simulink model "HubDepotModel"  (Simulink 7.9)
settings: Solver=VariableStepDiscrete  StartTime=0.0  StopTime=100.0  RelTol=1e-3
undefined symbols (not defined in the file or in its folder): CustomerBase_1
libraries: simeventslib x10
(part 2 of 4)

== system HubDepotModel/Depot_3/Storage_Subsystem/<<SOURCE>> Source_Stocked_Product ==
  Output Switch : OutputSwitch  NumberOutputPorts=2
  Path Combiner : PathCombiner  NumberInputPorts=2
  Schedule_Product_Deliveries_CONTROL : Subsystem
  Transfer_Product_CONTROL : Subsystem
  sS1.1_Schedule_Product_Deliveries_PLANT : Subsystem
  sS1.2_Receive_Product_PLANT : Subsystem
  sS1.3_Transfer_Product_PLANT : Subsystem
  sS1.3_Verify_Product_PLANT : Subsystem
  Inventory_IN : PMIOPort  Port=1  Side=Left
  Inventory_OUT : PMIOPort  Port=2  Side=Right
  Replenishment_Shipment : PMIOPort  Port=3  Side=Left
  Replenishment_Signal : PMIOPort  Port=4  Side=Left
  Procurement_Order : PMIOPort  Port=5  Side=Right
  wires:
  Schedule_Product_Deliveries_CONTROL/3(Reorder_Signal) -> sS1.1_Schedule_Product_Deliveries_PLANT/3(Reorder_Signal)
  Schedule_Product_Deliveries_CONTROL/1(Component) -> sS1.1_Schedule_Product_Deliveries_PLANT/1(Component)
  Schedule_Product_Deliveries_CONTROL/2(Reorder_Quantity) -> sS1.1_Schedule_Product_Deliveries_PLANT/2(Reorder_Quantity)
  connections:
  Replenishment_Signal/RConn1 -- Schedule_Product_Deliveries_CONTROL/LConn2
  Path Combiner/LConn1 -- Schedule_Product_Deliveries_CONTROL/RConn1
  Path Combiner/LConn2 -- Transfer_Product_CONTROL/RConn1
  Path Combiner/RConn1 -- Inventory_OUT/RConn1
  Output Switch/RConn2 -- Transfer_Product_CONTROL/LConn1
  Output Switch/RConn1 -- Schedule_Product_Deliveries_CONTROL/LConn1
  Inventory_IN/RConn1 -- Output Switch/LConn1
  sS1.1_Schedule_Product_Deliveries_PLANT/RConn1 -- Procurement_Order/RConn1
  sS1.3_Transfer_Product_PLANT/RConn1 -- Transfer_Product_CONTROL/LConn2
  sS1.3_Verify_Product_PLANT/RConn1 -- sS1.3_Transfer_Product_PLANT/LConn1
  sS1.2_Receive_Product_PLANT/RConn1 -- sS1.3_Verify_Product_PLANT/LConn1
  Replenishment_Shipment/RConn1 -- sS1.2_Receive_Product_PLANT/LConn1

== system HubDepotModel/Depot_4/Storage_Subsystem/<<DELIVER>>Deliver_Stocked_Product ==
  Deliver_Stocked_Product_CONTROL : Subsystem
  sD1.10_Pack_Order_PLANT : Subsystem
  sD1.11_Load_Order_PLANT : Subsystem
  sD1.2_Receive_Order_PLANT : Subsystem
  sD1.4_Consolidate_Orders_PLANT : Subsystem
  sD1.9_Pick_Order_PLANT : Subsystem
  Inventory_IN : PMIOPort  Port=1  Side=Left
  Inventory_OUT : PMIOPort  Port=2  Side=Right
  Customer_Procurement_Order : PMIOPort  Port=3  Side=Left
  Fulfillment_Shipment : PMIOPort  Port=4  Side=Right
  Replenishment_Signal : PMIOPort  Port=5  Side=Right
  connections:
  sD1.4_Consolidate_Orders_PLANT/RConn1 -- sD1.9_Pick_Order_PLANT/LConn1
  sD1.2_Receive_Order_PLANT/RConn1 -- sD1.4_Consolidate_Orders_PLANT/LConn1
  Deliver_Stocked_Product_CONTROL/RConn2 -- Inventory_OUT/RConn1
  Deliver_Stocked_Product_CONTROL/RConn1 -- Replenishment_Signal/RConn1
  Deliver_Stocked_Product_CONTROL/LConn1 -- Inventory_IN/RConn1
  sD1.9_Pick_Order_PLANT/RConn1 -- Deliver_Stocked_Product_CONTROL/LConn2
  sD1.11_Load_Order_PLANT/RConn1 -- Fulfillment_Shipment/RConn1
  sD1.10_Pack_Order_PLANT/RConn1 -- sD1.11_Load_Order_PLANT/LConn1
  sD1.9_Pick_Order_PLANT/RConn2 -- sD1.10_Pack_Order_PLANT/LConn1
  Customer_Procurement_Order/RConn1 -- sD1.2_Receive_Order_PLANT/LConn1

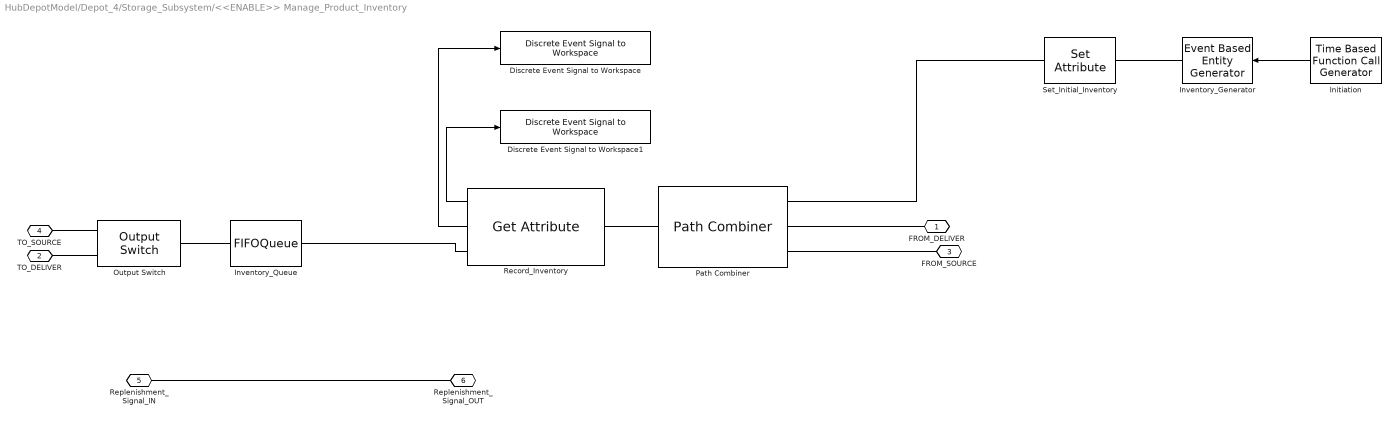
== system HubDepotModel/Depot_4/Storage_Subsystem/<<ENABLE>> Manage_Product_Inventory ==
  Discrete Event Signal to Workspace : simeventslib/SimEvents Sinks/Discrete Event Signal to Workspace  VariableName=Inventory_Position_Depot_1  SaveFormat=Structure With Time  isMonitorOnly=off  isRecordIC=off
  Discrete Event Signal to Workspace1 : simeventslib/SimEvents Sinks/Discrete Event Signal to Workspace  VariableName=Net_Inventory_Depot_1  SaveFormat=Structure With Time  isMonitorOnly=off  isRecordIC=off
  Initiation : TimeBasedFunctionCallGenerator  EventGenerationMode=Only at simulation start  EventPriority=1
  Inventory_Generator : EventBasedEntityGenerator  GenerateEntitiesUpon=Function call from port fcn  SpecifyEventPriority=on  PriorityEntityGeneration=1  AllowBlocking=off  EntityType=Standard
  Inventory_Queue : FIFOQueue
  Output Switch : OutputSwitch  NumberOutputPorts=2
  Path Combiner : PathCombiner
  Record_Inventory : GetAttribute  AttributeName=Net_Inventory|Inventory_Position  AttributeMissing=Error|Error  AttributeDefaultValue=1|1  AttributeTreatAsVector=1|1  AttributeSendTiming=After entity departure|After entity departure  EvaluatedDefaultAttributeValue={[];[]}
      settings: OutputPortMap=o1,o2
  Set_Initial_Inventory : SetAttribute  AttributeName=Net_Inventory|Inventory_Position|Reorder_Point|Reorder_Quantity  AttributeFrom=Dialog|Dialog|Dialog|Dialog  AttributeValue=[11 13]|[11 13]|[10 10]|[5 5]  AttributeTreatAsVector=1|1|1|1  EvaluatedAttributeValue={[11 13];[11 13];[10 10];[5 5]}
  FROM_DELIVER : PMIOPort  Port=1  Side=Left
  TO_DELIVER : PMIOPort  Port=2  Side=Right
  FROM_SOURCE : PMIOPort  Port=3  Side=Left
  TO_SOURCE : PMIOPort  Port=4  Side=Right
  Replenishment_Signal_IN : PMIOPort  Port=5  Side=Left
  Replenishment_Signal_OUT : PMIOPort  Port=6  Side=Right
  wires:
  Record_Inventory/2 -> Discrete Event Signal to Workspace/1
  Initiation/1 -> Inventory_Generator/1
  Record_Inventory/1 -> Discrete Event Signal to Workspace1/1
  connections:
  Set_Initial_Inventory/RConn1 -- Path Combiner/LConn1
  Replenishment_Signal_IN/RConn1 -- Replenishment_Signal_OUT/RConn1
  TO_SOURCE/RConn1 -- Output Switch/RConn1
  TO_DELIVER/RConn1 -- Output Switch/RConn2
  FROM_SOURCE/RConn1 -- Path Combiner/LConn3
  FROM_DELIVER/RConn1 -- Path Combiner/LConn2
  Record_Inventory/LConn1 -- Path Combiner/RConn1
  Output Switch/LConn1 -- Inventory_Queue/RConn1
  Record_Inventory/RConn1 -- Inventory_Queue/LConn1
  Set_Initial_Inventory/LConn1 -- Inventory_Generator/RConn1

== system HubDepotModel/Depot_4/Storage_Subsystem/<<SOURCE>> Source_Stocked_Product ==
  Output Switch : OutputSwitch  NumberOutputPorts=2
  Path Combiner : PathCombiner  NumberInputPorts=2
  Schedule_Product_Deliveries_CONTROL : Subsystem
  Transfer_Product_CONTROL : Subsystem
  sS1.1_Schedule_Product_Deliveries_PLANT : Subsystem
  sS1.2_Receive_Product_PLANT : Subsystem
  sS1.3_Transfer_Product_PLANT : Subsystem
  sS1.3_Verify_Product_PLANT : Subsystem
  Inventory_IN : PMIOPort  Port=1  Side=Left
  Inventory_OUT : PMIOPort  Port=2  Side=Right
  Replenishment_Shipment : PMIOPort  Port=3  Side=Left
  Replenishment_Signal : PMIOPort  Port=4  Side=Left
  Procurement_Order : PMIOPort  Port=5  Side=Right
  wires:
  Schedule_Product_Deliveries_CONTROL/3(Reorder_Signal) -> sS1.1_Schedule_Product_Deliveries_PLANT/3(Reorder_Signal)
  Schedule_Product_Deliveries_CONTROL/1(Component) -> sS1.1_Schedule_Product_Deliveries_PLANT/1(Component)
  Schedule_Product_Deliveries_CONTROL/2(Reorder_Quantity) -> sS1.1_Schedule_Product_Deliveries_PLANT/2(Reorder_Quantity)
  connections:
  Replenishment_Signal/RConn1 -- Schedule_Product_Deliveries_CONTROL/LConn2
  Path Combiner/LConn1 -- Schedule_Product_Deliveries_CONTROL/RConn1
  Path Combiner/LConn2 -- Transfer_Product_CONTROL/RConn1
  Path Combiner/RConn1 -- Inventory_OUT/RConn1
  Output Switch/RConn2 -- Transfer_Product_CONTROL/LConn1
  Output Switch/RConn1 -- Schedule_Product_Deliveries_CONTROL/LConn1
  Inventory_IN/RConn1 -- Output Switch/LConn1
  sS1.1_Schedule_Product_Deliveries_PLANT/RConn1 -- Procurement_Order/RConn1
  sS1.3_Transfer_Product_PLANT/RConn1 -- Transfer_Product_CONTROL/LConn2
  sS1.3_Verify_Product_PLANT/RConn1 -- sS1.3_Transfer_Product_PLANT/LConn1
  sS1.2_Receive_Product_PLANT/RConn1 -- sS1.3_Verify_Product_PLANT/LConn1
  Replenishment_Shipment/RConn1 -- sS1.2_Receive_Product_PLANT/LConn1

== system HubDepotModel/Hub_1/Storage_Subsystem/<<DELIVER>>Deliver_Stocked_Product ==
  Deliver_Stocked_Product_CONTROL : Subsystem
  sD1.10_Pack_Order_PLANT : Subsystem
  sD1.11_Load_Order_PLANT : Subsystem
  sD1.2_Receive_Order_PLANT : Subsystem
  sD1.4_Consolidate_Orders_PLANT : Subsystem
  sD1.9_Pick_Order_PLANT : Subsystem
  Inventory_IN : PMIOPort  Port=1  Side=Left
  Inventory_OUT : PMIOPort  Port=2  Side=Right
  Customer_Procurement_Order : PMIOPort  Port=3  Side=Left
  Fulfillment_Shipment : PMIOPort  Port=4  Side=Right
  Replenishment_Signal : PMIOPort  Port=5  Side=Right
  connections:
  sD1.4_Consolidate_Orders_PLANT/RConn1 -- sD1.9_Pick_Order_PLANT/LConn1
  sD1.2_Receive_Order_PLANT/RConn1 -- sD1.4_Consolidate_Orders_PLANT/LConn1
  Deliver_Stocked_Product_CONTROL/RConn2 -- Inventory_OUT/RConn1
  Deliver_Stocked_Product_CONTROL/RConn1 -- Replenishment_Signal/RConn1
  Deliver_Stocked_Product_CONTROL/LConn1 -- Inventory_IN/RConn1
  sD1.9_Pick_Order_PLANT/RConn1 -- Deliver_Stocked_Product_CONTROL/LConn2
  sD1.11_Load_Order_PLANT/RConn1 -- Fulfillment_Shipment/RConn1
  sD1.10_Pack_Order_PLANT/RConn1 -- sD1.11_Load_Order_PLANT/LConn1
  sD1.9_Pick_Order_PLANT/RConn2 -- sD1.10_Pack_Order_PLANT/LConn1
  Customer_Procurement_Order/RConn1 -- sD1.2_Receive_Order_PLANT/LConn1

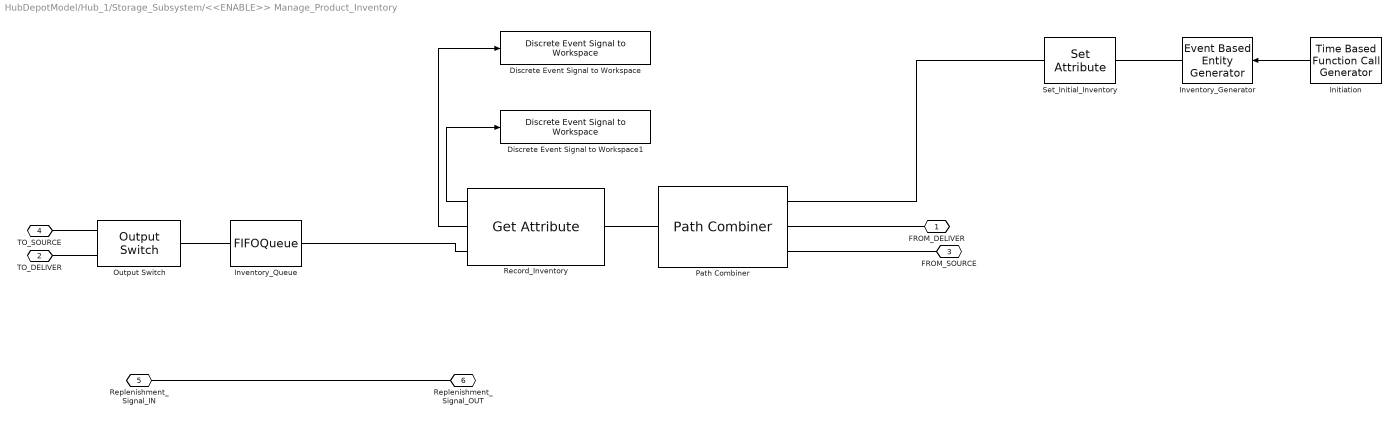
== system HubDepotModel/Hub_1/Storage_Subsystem/<<ENABLE>> Manage_Product_Inventory ==
  Discrete Event Signal to Workspace : simeventslib/SimEvents Sinks/Discrete Event Signal to Workspace  VariableName=Inventory_Position_Depot_1  SaveFormat=Structure With Time  isMonitorOnly=off  isRecordIC=off
  Discrete Event Signal to Workspace1 : simeventslib/SimEvents Sinks/Discrete Event Signal to Workspace  VariableName=Net_Inventory_Depot_1  SaveFormat=Structure With Time  isMonitorOnly=off  isRecordIC=off
  Initiation : TimeBasedFunctionCallGenerator  EventGenerationMode=Only at simulation start  EventPriority=1
  Inventory_Generator : EventBasedEntityGenerator  GenerateEntitiesUpon=Function call from port fcn  SpecifyEventPriority=on  PriorityEntityGeneration=1  AllowBlocking=off  EntityType=Standard
  Inventory_Queue : FIFOQueue
  Output Switch : OutputSwitch  NumberOutputPorts=2
  Path Combiner : PathCombiner
  Record_Inventory : GetAttribute  AttributeName=Net_Inventory|Inventory_Position  AttributeMissing=Error|Error  AttributeDefaultValue=1|1  AttributeTreatAsVector=1|1  AttributeSendTiming=After entity departure|After entity departure  EvaluatedDefaultAttributeValue={[];[]}
      settings: OutputPortMap=o1,o2
  Set_Initial_Inventory : SetAttribute  AttributeName=Net_Inventory|Inventory_Position|Reorder_Point|Reorder_Quantity  AttributeFrom=Dialog|Dialog|Dialog|Dialog  AttributeValue=[11 13]|[11 13]|[10 10]|[5 5]  AttributeTreatAsVector=1|1|1|1  EvaluatedAttributeValue={[11 13];[11 13];[10 10];[5 5]}
  FROM_DELIVER : PMIOPort  Port=1  Side=Left
  TO_DELIVER : PMIOPort  Port=2  Side=Right
  FROM_SOURCE : PMIOPort  Port=3  Side=Left
  TO_SOURCE : PMIOPort  Port=4  Side=Right
  Replenishment_Signal_IN : PMIOPort  Port=5  Side=Left
  Replenishment_Signal_OUT : PMIOPort  Port=6  Side=Right
  wires:
  Record_Inventory/2 -> Discrete Event Signal to Workspace/1
  Initiation/1 -> Inventory_Generator/1
  Record_Inventory/1 -> Discrete Event Signal to Workspace1/1
  connections:
  Set_Initial_Inventory/RConn1 -- Path Combiner/LConn1
  Replenishment_Signal_IN/RConn1 -- Replenishment_Signal_OUT/RConn1
  TO_SOURCE/RConn1 -- Output Switch/RConn1
  TO_DELIVER/RConn1 -- Output Switch/RConn2
  FROM_SOURCE/RConn1 -- Path Combiner/LConn3
  FROM_DELIVER/RConn1 -- Path Combiner/LConn2
  Record_Inventory/LConn1 -- Path Combiner/RConn1
  Output Switch/LConn1 -- Inventory_Queue/RConn1
  Record_Inventory/RConn1 -- Inventory_Queue/LConn1
  Set_Initial_Inventory/LConn1 -- Inventory_Generator/RConn1

== system HubDepotModel/Hub_1/Storage_Subsystem/<<SOURCE>> Source_Stocked_Product ==
  Output Switch : OutputSwitch  NumberOutputPorts=2
  Path Combiner : PathCombiner  NumberInputPorts=2
  Schedule_Product_Deliveries_CONTROL : Subsystem
  Transfer_Product_CONTROL : Subsystem
  sS1.1_Schedule_Product_Deliveries_PLANT : Subsystem
  sS1.2_Receive_Product_PLANT : Subsystem
  sS1.3_Transfer_Product_PLANT : Subsystem
  sS1.3_Verify_Product_PLANT : Subsystem
  Inventory_IN : PMIOPort  Port=1  Side=Left
  Inventory_OUT : PMIOPort  Port=2  Side=Right
  Replenishment_Shipment : PMIOPort  Port=3  Side=Left
  Replenishment_Signal : PMIOPort  Port=4  Side=Left
  Procurement_Order : PMIOPort  Port=5  Side=Right
  wires:
  Schedule_Product_Deliveries_CONTROL/3(Reorder_Signal) -> sS1.1_Schedule_Product_Deliveries_PLANT/3(Reorder_Signal)
  Schedule_Product_Deliveries_CONTROL/1(Component) -> sS1.1_Schedule_Product_Deliveries_PLANT/1(Component)
  Schedule_Product_Deliveries_CONTROL/2(Reorder_Quantity) -> sS1.1_Schedule_Product_Deliveries_PLANT/2(Reorder_Quantity)
  connections:
  Replenishment_Signal/RConn1 -- Schedule_Product_Deliveries_CONTROL/LConn2
  Path Combiner/LConn1 -- Schedule_Product_Deliveries_CONTROL/RConn1
  Path Combiner/LConn2 -- Transfer_Product_CONTROL/RConn1
  Path Combiner/RConn1 -- Inventory_OUT/RConn1
  Output Switch/RConn2 -- Transfer_Product_CONTROL/LConn1
  Output Switch/RConn1 -- Schedule_Product_Deliveries_CONTROL/LConn1
  Inventory_IN/RConn1 -- Output Switch/LConn1
  sS1.1_Schedule_Product_Deliveries_PLANT/RConn1 -- Procurement_Order/RConn1
  sS1.3_Transfer_Product_PLANT/RConn1 -- Transfer_Product_CONTROL/LConn2
  sS1.3_Verify_Product_PLANT/RConn1 -- sS1.3_Transfer_Product_PLANT/LConn1
  sS1.2_Receive_Product_PLANT/RConn1 -- sS1.3_Verify_Product_PLANT/LConn1
  Replenishment_Shipment/RConn1 -- sS1.2_Receive_Product_PLANT/LConn1

== system HubDepotModel/Depot_1/Storage_Subsystem/<<DELIVER>>Deliver_Stocked_Product/Deliver_Stocked_Product_CONTROL ==
  Calculate_Inventory_C : MATLAB Function  TreatAsAtomicUnit=on
  Combine_Consumption_Inventory : EntityCombiner  NumberInputPorts=2
  Consumption_Attributes : GetAttribute  AttributeName=Component|Consumption_Quantity|Net_Inventory|Inventory_Position  AttributeMissing=Error|Error|Error|Error  AttributeDefaultValue=1|1|1|1  AttributeTreatAsVector=1|1|1|1  AttributeSendTiming=After entity departure|After entity departure|After entity departure|After entity departure  EvaluatedDefaultAttributeValue={[];[];[];[]}
      settings: OutputPortMap=o1,o2,o3,o4
  Consumption_Server : SingleServer  ServiceTime=0
  Consumption_Sink : EntitySink
  FIFO Queue : FIFOQueue
  Replicate : Replicate  NumberOutputPorts=2
  Return_Inventory : EntitySplitter  NumberOutputPorts=2
  Set_Inventory_Level : SetAttribute  AttributeName=Net_Inventory|Inventory_Position  AttributeFrom=Signal port|Signal port  AttributeValue=1|1  AttributeTreatAsVector=1|1  EvaluatedAttributeValue={[];[]}
      settings: InputPortMap=u0,u1
  Inventory_IN : PMIOPort  Port=1  Side=Left
  Consumption_Signal_IN : PMIOPort  Port=2  Side=Left
  Consumption_Signal_OUT : PMIOPort  Port=3  Side=Right
  Inventory_OUT : PMIOPort  Port=4  Side=Right
  wires:
  Calculate_Inventory_C/2(out_Inventory_Position) -> Set_Inventory_Level/2
  Consumption_Attributes/4 -> Calculate_Inventory_C/2(Inventory_Position)
  Consumption_Attributes/2 -> Calculate_Inventory_C/4(Consumption_Quantity)
  Consumption_Attributes/3 -> Calculate_Inventory_C/1(Net_Inventory)
  Calculate_Inventory_C/1(out_Net_Inventory) -> Set_Inventory_Level/1
  Consumption_Attributes/1 -> Calculate_Inventory_C/3(Component)
  connections:
  Inventory_OUT/RConn1 -- Return_Inventory/RConn1
  Set_Inventory_Level/RConn1 -- Return_Inventory/LConn1
  Replicate/RConn2 -- Consumption_Signal_OUT/RConn1
  Return_Inventory/RConn2 -- Consumption_Sink/LConn1
  Consumption_Server/RConn1 -- Set_Inventory_Level/LConn1
  Consumption_Attributes/RConn1 -- Consumption_Server/LConn1
  Combine_Consumption_Inventory/RConn1 -- Consumption_Attributes/LConn1
  Replicate/RConn1 -- Combine_Consumption_Inventory/LConn2
  Inventory_IN/RConn1 -- Combine_Consumption_Inventory/LConn1
  Consumption_Signal_IN/RConn1 -- FIFO Queue/LConn1
  FIFO Queue/RConn1 -- Replicate/LConn1

== system HubDepotModel/Depot_1/Storage_Subsystem/<<DELIVER>>Deliver_Stocked_Product/sD1.10_Pack_Order_PLANT ==
  Entity Departure Function-Call Generator : EntityDepartureFunctionCallGenerator
  Event-Based Entity Generator : EventBasedEntityGenerator  GenerateEntitiesUpon=Function call from port fcn
  Get_Order_Attribute : GetAttribute  AttributeName=Component|Order_Quantity|Customer  AttributeMissing=Error|Error|Error  AttributeDefaultValue=1|1|1  AttributeTreatAsVector=1|1|1  AttributeSendTiming=After entity departure|After entity departure|After entity departure  EvaluatedDefaultAttributeValue={[];[];[]}
      settings: OutputPortMap=o1,o2,o3
  Order_Sink : EntitySink
  Set_Shipment_Attributes : SetAttribute  AttributeName=Component|Shipment_Quantity|Customer  AttributeFrom=Signal port|Signal port|Signal port  AttributeValue=1|1|1  AttributeTreatAsVector=1|1|1  EvaluatedAttributeValue={[];[];[]}
      settings: InputPortMap=u0,u1,u2
  sD1.10_Queue : FIFOQueue
  sD1.10_Server : NServer  NumberOfServers=inf  ServiceTime=0
  Order_IN : PMIOPort  Port=1  Side=Left
  Shipment_OUT : PMIOPort  Port=2  Side=Right
  wires:
  Get_Order_Attribute/3 -> Set_Shipment_Attributes/3
  Get_Order_Attribute/1 -> Set_Shipment_Attributes/1
  Get_Order_Attribute/2 -> Set_Shipment_Attributes/2
  Entity Departure Function-Call Generator/1 -> Event-Based Entity Generator/1
  connections:
  Get_Order_Attribute/RConn1 -- Entity Departure Function-Call Generator/LConn1
  sD1.10_Server/RConn1 -- Get_Order_Attribute/LConn1
  Order_Sink/LConn1 -- Entity Departure Function-Call Generator/RConn1
  Set_Shipment_Attributes/RConn1 -- Shipment_OUT/RConn1
  Event-Based Entity Generator/RConn1 -- Set_Shipment_Attributes/LConn1
  Order_IN/RConn1 -- sD1.10_Queue/LConn1
  sD1.10_Queue/RConn1 -- sD1.10_Server/LConn1

== system HubDepotModel/Depot_1/Storage_Subsystem/<<DELIVER>>Deliver_Stocked_Product/sD1.11_Load_Order_PLANT ==
  sD1.11_Queue : FIFOQueue
  sD1.11_Server : NServer  NumberOfServers=inf  ServiceTime=0
  Shipment_IN : PMIOPort  Port=1  Side=Left
  Shipment_OUT : PMIOPort  Port=2  Side=Right
  connections:
  Shipment_OUT/RConn1 -- sD1.11_Server/RConn1
  Shipment_IN/RConn1 -- sD1.11_Queue/LConn1
  sD1.11_Queue/RConn1 -- sD1.11_Server/LConn1

== system HubDepotModel/Depot_1/Storage_Subsystem/<<DELIVER>>Deliver_Stocked_Product/sD1.2_Receive_Order_PLANT ==
  sD1.2_Queue : FIFOQueue
  sD1.2_Server : NServer  NumberOfServers=inf  ServiceTime=0
  Order_IN : PMIOPort  Port=1  Side=Left
  Order_OUT : PMIOPort  Port=2  Side=Right
  connections:
  Order_OUT/RConn1 -- sD1.2_Server/RConn1
  Order_IN/RConn1 -- sD1.2_Queue/LConn1
  sD1.2_Queue/RConn1 -- sD1.2_Server/LConn1

== system HubDepotModel/Depot_1/Storage_Subsystem/<<DELIVER>>Deliver_Stocked_Product/sD1.4_Consolidate_Orders_PLANT ==
  sD1.4_Queue : FIFOQueue
  sD1.4_Server : NServer  NumberOfServers=inf  ServiceTime=0
  Order_IN : PMIOPort  Port=1  Side=Left
  Order_OUT : PMIOPort  Port=2  Side=Right
  connections:
  Order_OUT/RConn1 -- sD1.4_Server/RConn1
  Order_IN/RConn1 -- sD1.4_Queue/LConn1
  sD1.4_Queue/RConn1 -- sD1.4_Server/LConn1

== system HubDepotModel/Depot_1/Storage_Subsystem/<<DELIVER>>Deliver_Stocked_Product/sD1.9_Pick_Order_PLANT ==
  Generate_Consumption_Signal : Subsystem
  sD1.9_Queue : FIFOQueue
  sD1.9_Server : NServer  NumberOfServers=inf  ServiceTime=0
  Order_IN : PMIOPort  Port=1  Side=Left
  Consumption_Signal : PMIOPort  Port=2  Side=Right
  Order_OUT : PMIOPort  Port=3  Side=Right
  connections:
  Generate_Consumption_Signal/RConn2 -- Consumption_Signal/RConn1
  Generate_Consumption_Signal/RConn1 -- Order_OUT/RConn1
  sD1.9_Server/RConn1 -- Generate_Consumption_Signal/LConn1
  Order_IN/RConn1 -- sD1.9_Queue/LConn1
  sD1.9_Queue/RConn1 -- sD1.9_Server/LConn1

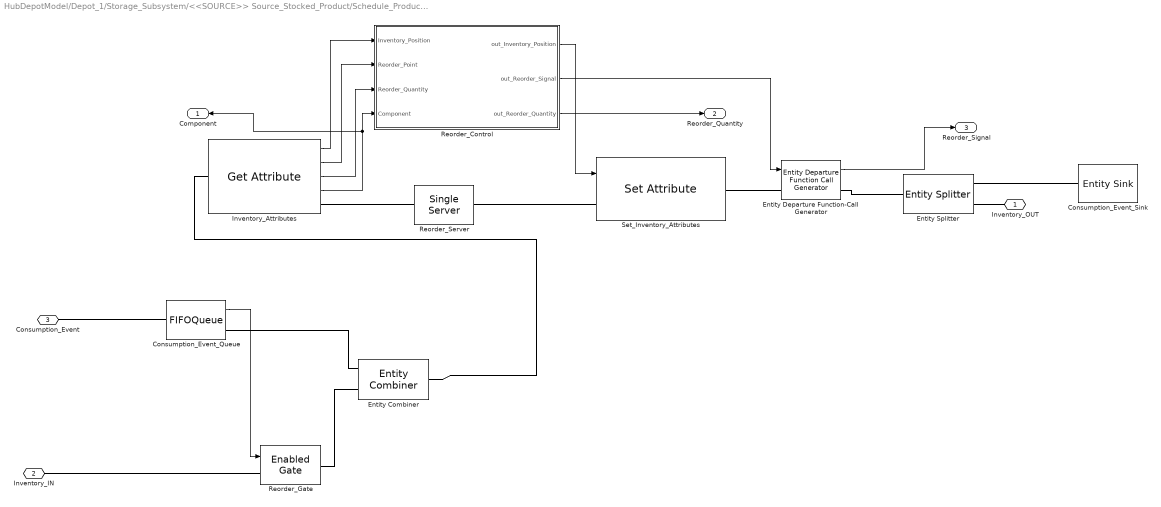
== system HubDepotModel/Depot_1/Storage_Subsystem/<<SOURCE>> Source_Stocked_Product/Schedule_Product_Deliveries_CONTROL ==
  Consumption_Event_Queue : FIFOQueue  StatNumberInBlock=on
      settings: OutputPortMap=o1
  Consumption_Event_Sink : EntitySink
  Entity Combiner : EntityCombiner  NumberInputPorts=2
  Entity Departure Function-Call Generator : EntityDepartureFunctionCallGenerator  EnableE1Port=on
  Entity Splitter : EntitySplitter  NumberOutputPorts=2
  Inventory_Attributes : GetAttribute  AttributeName=Inventory_Position|Reorder_Point|Reorder_Quantity|Component  AttributeMissing=Error|Error|Error|Error  AttributeDefaultValue=1|1|1|1  AttributeTreatAsVector=1|1|1|1  AttributeSendTiming=After entity departure|After entity departure|After entity departure|After entity departure  EvaluatedDefaultAttributeValue={[];[];[];[]}
      settings: OutputPortMap=o1,o2,o3,o4
  Reorder_Control : MATLAB Function  TreatAsAtomicUnit=on
  Reorder_Gate : EnabledGate
  Reorder_Server : SingleServer  ServiceTime=0
  Set_Inventory_Attributes : SetAttribute  AttributeName=Inventory_Position  AttributeFrom=Signal port  EvaluatedAttributeValue={[]}
  Inventory_OUT : PMIOPort  Port=1  Side=Right
  Inventory_IN : PMIOPort  Port=2  Side=Left
  Consumption_Event : PMIOPort  Port=3  Side=Left
  Component : Outport
  Reorder_Quantity : Outport  Port=2
  Reorder_Signal : Outport  Port=3
  wires:
  Entity Departure Function-Call Generator/1 -> Reorder_Signal/1
  Reorder_Control/3(out_Reorder_Quantity) -> Reorder_Quantity/1
  Consumption_Event_Queue/1 -> Reorder_Gate/1
  Reorder_Control/2(out_Reorder_Signal) -> Entity Departure Function-Call Generator/1
  Inventory_Attributes/4 -> Component/1, Reorder_Control/4(Component)
  Reorder_Control/1(out_Inventory_Position) -> Set_Inventory_Attributes/1
  Inventory_Attributes/3 -> Reorder_Control/3(Reorder_Quantity)
  Inventory_Attributes/2 -> Reorder_Control/2(Reorder_Point)
  Inventory_Attributes/1 -> Reorder_Control/1(Inventory_Position)
  connections:
  Entity Departure Function-Call Generator/RConn1 -- Entity Splitter/LConn1
  Set_Inventory_Attributes/RConn1 -- Entity Departure Function-Call Generator/LConn1
  Reorder_Server/RConn1 -- Set_Inventory_Attributes/LConn1
  Inventory_IN/RConn1 -- Reorder_Gate/LConn1
  Inventory_Attributes/RConn1 -- Reorder_Server/LConn1
  Inventory_OUT/RConn1 -- Entity Splitter/RConn2
  Entity Combiner/RConn1 -- Inventory_Attributes/LConn1
  Reorder_Gate/RConn1 -- Entity Combiner/LConn2
  Entity Splitter/RConn1 -- Consumption_Event_Sink/LConn1
  Consumption_Event_Queue/RConn1 -- Entity Combiner/LConn1
  Consumption_Event/RConn1 -- Consumption_Event_Queue/LConn1

== system HubDepotModel/Depot_1/Storage_Subsystem/<<SOURCE>> Source_Stocked_Product/Transfer_Product_CONTROL ==
  Calculate_Inventory : MATLAB Function  TreatAsAtomicUnit=on
  Combine_Inventory_and_Availability : EntityCombiner  NumberInputPorts=2
  FIFO Queue : FIFOQueue
  Inventory_Availability_Attributes : GetAttribute  AttributeName=Component|Shipment_Quantity|Net_Inventory  AttributeMissing=Error|Error|Error  AttributeDefaultValue=1|1|1  AttributeTreatAsVector=1|1|1  AttributeSendTiming=After entity departure|After entity departure|After entity departure  EvaluatedDefaultAttributeValue={[];[];[]}
      settings: OutputPortMap=o1,o2,o3
  Inventory_Availability_Sink : EntitySink
  Return_Inventory : EntitySplitter  NumberOutputPorts=2
  Server : SingleServer  ServiceTime=0
  Set_Inventory_Level : SetAttribute  AttributeName=Net_Inventory  AttributeFrom=Signal port  EvaluatedAttributeValue={[]}
  Inventory_OUT : PMIOPort  Port=1  Side=Right
  Inventory_IN : PMIOPort  Port=2  Side=Left
  Inventory_Availability_Signal : PMIOPort  Port=3  Side=Left
  wires:
  Inventory_Availability_Attributes/2 -> Calculate_Inventory/3(Shipment_Quantity)
  Inventory_Availability_Attributes/3 -> Calculate_Inventory/1(Net_Inventory)
  Calculate_Inventory/1(out_Inventory) -> Set_Inventory_Level/1
  Inventory_Availability_Attributes/1 -> Calculate_Inventory/2(Component)
  connections:
  Inventory_IN/RConn1 -- Combine_Inventory_and_Availability/LConn1
  FIFO Queue/RConn1 -- Combine_Inventory_and_Availability/LConn2
  Inventory_Availability_Signal/RConn1 -- FIFO Queue/LConn1
  Inventory_OUT/RConn1 -- Return_Inventory/RConn1
  Set_Inventory_Level/RConn1 -- Return_Inventory/LConn1
  Return_Inventory/RConn2 -- Inventory_Availability_Sink/LConn1
  Server/RConn1 -- Set_Inventory_Level/LConn1
  Inventory_Availability_Attributes/RConn1 -- Server/LConn1
  Combine_Inventory_and_Availability/RConn1 -- Inventory_Availability_Attributes/LConn1

== system HubDepotModel/Depot_1/Storage_Subsystem/<<SOURCE>> Source_Stocked_Product/sS1.1_Schedule_Product_Deliveries_PLANT ==
  Component : Inport
  Reorder_Quantity : Inport  Port=2
  Reorder_Signal : Inport  Port=3
  Generate_Procurement_Order : Subsystem
  Schedule_Product_Deliveries_Server : NServer  NumberOfServers=inf  ServiceTime=0
  Set_Procurement_Order : SetAttribute  AttributeName=Component|Order_Quantity|Supplier|Customer  AttributeFrom=Signal port|Signal port|Dialog|Dialog  AttributeValue=1|1|1|1  AttributeTreatAsVector=1|1|1|1  EvaluatedAttributeValue={[];[];1;1}
      settings: InputPortMap=u0,u1
  Procurement_Order : PMIOPort  Port=1  Side=Right
  wires:
  Reorder_Signal/1 -> Generate_Procurement_Order/1(Reorder_Signal)
  Reorder_Quantity/1 -> Set_Procurement_Order/2
  Component/1 -> Set_Procurement_Order/1
  connections:
  Procurement_Order/RConn1 -- Set_Procurement_Order/RConn1
  Schedule_Product_Deliveries_Server/RConn1 -- Set_Procurement_Order/LConn1
  Generate_Procurement_Order/RConn1 -- Schedule_Product_Deliveries_Server/LConn1

== system HubDepotModel/Depot_1/Storage_Subsystem/<<SOURCE>> Source_Stocked_Product/sS1.2_Receive_Product_PLANT ==
  sS1.2_Queue : FIFOQueue  Capacity=inf
  sS1.2_Server : NServer  NumberOfServers=inf  ServiceTime=0
  Shipment_IN : PMIOPort  Port=1  Side=Left
  Component_OUT : PMIOPort  Port=2  Side=Right
  connections:
  Component_OUT/RConn1 -- sS1.2_Server/RConn1
  Shipment_IN/RConn1 -- sS1.2_Queue/LConn1
  sS1.2_Queue/RConn1 -- sS1.2_Server/LConn1

== system HubDepotModel/Depot_1/Storage_Subsystem/<<SOURCE>> Source_Stocked_Product/sS1.3_Transfer_Product_PLANT ==
  sS1.4_Queue : FIFOQueue
  sS1.4_Server : NServer  NumberOfServers=inf  ServiceTime=0
  Component_IN : PMIOPort  Port=1  Side=Left
  Inventory_Availability_Signal : PMIOPort  Port=2  Side=Right
  connections:
  Inventory_Availability_Signal/RConn1 -- sS1.4_Server/RConn1
  Component_IN/RConn1 -- sS1.4_Queue/LConn1
  sS1.4_Queue/RConn1 -- sS1.4_Server/LConn1

== system HubDepotModel/Depot_1/Storage_Subsystem/<<SOURCE>> Source_Stocked_Product/sS1.3_Verify_Product_PLANT ==
  sS1.3_Queue : FIFOQueue  Capacity=inf
  sS1.3_Server : NServer  NumberOfServers=inf  ServiceTime=0
  Component_IN : PMIOPort  Port=1  Side=Left
  Component_OUT : PMIOPort  Port=2  Side=Right
  connections:
  Component_OUT/RConn1 -- sS1.3_Server/RConn1
  Component_IN/RConn1 -- sS1.3_Queue/LConn1
  sS1.3_Queue/RConn1 -- sS1.3_Server/LConn1

== system HubDepotModel/Depot_2/Storage_Subsystem/<<DELIVER>>Deliver_Stocked_Product/Deliver_Stocked_Product_CONTROL ==
  Calculate_Inventory_C : MATLAB Function  TreatAsAtomicUnit=on
  Combine_Consumption_Inventory : EntityCombiner  NumberInputPorts=2
  Consumption_Attributes : GetAttribute  AttributeName=Component|Consumption_Quantity|Net_Inventory|Inventory_Position  AttributeMissing=Error|Error|Error|Error  AttributeDefaultValue=1|1|1|1  AttributeTreatAsVector=1|1|1|1  AttributeSendTiming=After entity departure|After entity departure|After entity departure|After entity departure  EvaluatedDefaultAttributeValue={[];[];[];[]}
      settings: OutputPortMap=o1,o2,o3,o4
  Consumption_Server : SingleServer  ServiceTime=0
  Consumption_Sink : EntitySink
  FIFO Queue : FIFOQueue
  Replicate : Replicate  NumberOutputPorts=2
  Return_Inventory : EntitySplitter  NumberOutputPorts=2
  Set_Inventory_Level : SetAttribute  AttributeName=Net_Inventory|Inventory_Position  AttributeFrom=Signal port|Signal port  AttributeValue=1|1  AttributeTreatAsVector=1|1  EvaluatedAttributeValue={[];[]}
      settings: InputPortMap=u0,u1
  Inventory_IN : PMIOPort  Port=1  Side=Left
  Consumption_Signal_IN : PMIOPort  Port=2  Side=Left
  Consumption_Signal_OUT : PMIOPort  Port=3  Side=Right
  Inventory_OUT : PMIOPort  Port=4  Side=Right
  wires:
  Calculate_Inventory_C/2(out_Inventory_Position) -> Set_Inventory_Level/2
  Consumption_Attributes/4 -> Calculate_Inventory_C/2(Inventory_Position)
  Consumption_Attributes/2 -> Calculate_Inventory_C/4(Consumption_Quantity)
  Consumption_Attributes/3 -> Calculate_Inventory_C/1(Net_Inventory)
  Calculate_Inventory_C/1(out_Net_Inventory) -> Set_Inventory_Level/1
  Consumption_Attributes/1 -> Calculate_Inventory_C/3(Component)
  connections:
  Inventory_OUT/RConn1 -- Return_Inventory/RConn1
  Set_Inventory_Level/RConn1 -- Return_Inventory/LConn1
  Replicate/RConn2 -- Consumption_Signal_OUT/RConn1
  Return_Inventory/RConn2 -- Consumption_Sink/LConn1
  Consumption_Server/RConn1 -- Set_Inventory_Level/LConn1
  Consumption_Attributes/RConn1 -- Consumption_Server/LConn1
  Combine_Consumption_Inventory/RConn1 -- Consumption_Attributes/LConn1
  Replicate/RConn1 -- Combine_Consumption_Inventory/LConn2
  Inventory_IN/RConn1 -- Combine_Consumption_Inventory/LConn1
  Consumption_Signal_IN/RConn1 -- FIFO Queue/LConn1
  FIFO Queue/RConn1 -- Replicate/LConn1

== system HubDepotModel/Depot_2/Storage_Subsystem/<<DELIVER>>Deliver_Stocked_Product/sD1.10_Pack_Order_PLANT ==
  Entity Departure Function-Call Generator : EntityDepartureFunctionCallGenerator
  Event-Based Entity Generator : EventBasedEntityGenerator  GenerateEntitiesUpon=Function call from port fcn
  Get_Order_Attribute : GetAttribute  AttributeName=Component|Order_Quantity|Customer  AttributeMissing=Error|Error|Error  AttributeDefaultValue=1|1|1  AttributeTreatAsVector=1|1|1  AttributeSendTiming=After entity departure|After entity departure|After entity departure  EvaluatedDefaultAttributeValue={[];[];[]}
      settings: OutputPortMap=o1,o2,o3
  Order_Sink : EntitySink
  Set_Shipment_Attributes : SetAttribute  AttributeName=Component|Shipment_Quantity|Customer  AttributeFrom=Signal port|Signal port|Signal port  AttributeValue=1|1|1  AttributeTreatAsVector=1|1|1  EvaluatedAttributeValue={[];[];[]}
      settings: InputPortMap=u0,u1,u2
  sD1.10_Queue : FIFOQueue
  sD1.10_Server : NServer  NumberOfServers=inf  ServiceTime=0
  Order_IN : PMIOPort  Port=1  Side=Left
  Shipment_OUT : PMIOPort  Port=2  Side=Right
  wires:
  Get_Order_Attribute/3 -> Set_Shipment_Attributes/3
  Get_Order_Attribute/1 -> Set_Shipment_Attributes/1
  Get_Order_Attribute/2 -> Set_Shipment_Attributes/2
  Entity Departure Function-Call Generator/1 -> Event-Based Entity Generator/1
  connections:
  Get_Order_Attribute/RConn1 -- Entity Departure Function-Call Generator/LConn1
  sD1.10_Server/RConn1 -- Get_Order_Attribute/LConn1
  Order_Sink/LConn1 -- Entity Departure Function-Call Generator/RConn1
  Set_Shipment_Attributes/RConn1 -- Shipment_OUT/RConn1
  Event-Based Entity Generator/RConn1 -- Set_Shipment_Attributes/LConn1
  Order_IN/RConn1 -- sD1.10_Queue/LConn1
  sD1.10_Queue/RConn1 -- sD1.10_Server/LConn1

== system HubDepotModel/Depot_2/Storage_Subsystem/<<DELIVER>>Deliver_Stocked_Product/sD1.11_Load_Order_PLANT ==
  sD1.11_Queue : FIFOQueue
  sD1.11_Server : NServer  NumberOfServers=inf  ServiceTime=0
  Shipment_IN : PMIOPort  Port=1  Side=Left
  Shipment_OUT : PMIOPort  Port=2  Side=Right
  connections:
  Shipment_OUT/RConn1 -- sD1.11_Server/RConn1
  Shipment_IN/RConn1 -- sD1.11_Queue/LConn1
  sD1.11_Queue/RConn1 -- sD1.11_Server/LConn1

== system HubDepotModel/Depot_2/Storage_Subsystem/<<DELIVER>>Deliver_Stocked_Product/sD1.2_Receive_Order_PLANT ==
  sD1.2_Queue : FIFOQueue
  sD1.2_Server : NServer  NumberOfServers=inf  ServiceTime=0
  Order_IN : PMIOPort  Port=1  Side=Left
  Order_OUT : PMIOPort  Port=2  Side=Right
  connections:
  Order_OUT/RConn1 -- sD1.2_Server/RConn1
  Order_IN/RConn1 -- sD1.2_Queue/LConn1
  sD1.2_Queue/RConn1 -- sD1.2_Server/LConn1

== system HubDepotModel/Depot_2/Storage_Subsystem/<<DELIVER>>Deliver_Stocked_Product/sD1.4_Consolidate_Orders_PLANT ==
  sD1.4_Queue : FIFOQueue
  sD1.4_Server : NServer  NumberOfServers=inf  ServiceTime=0
  Order_IN : PMIOPort  Port=1  Side=Left
  Order_OUT : PMIOPort  Port=2  Side=Right
  connections:
  Order_OUT/RConn1 -- sD1.4_Server/RConn1
  Order_IN/RConn1 -- sD1.4_Queue/LConn1
  sD1.4_Queue/RConn1 -- sD1.4_Server/LConn1

== system HubDepotModel/Depot_2/Storage_Subsystem/<<DELIVER>>Deliver_Stocked_Product/sD1.9_Pick_Order_PLANT ==
  Generate_Consumption_Signal : Subsystem
  sD1.9_Queue : FIFOQueue
  sD1.9_Server : NServer  NumberOfServers=inf  ServiceTime=0
  Order_IN : PMIOPort  Port=1  Side=Left
  Consumption_Signal : PMIOPort  Port=2  Side=Right
  Order_OUT : PMIOPort  Port=3  Side=Right
  connections:
  Generate_Consumption_Signal/RConn2 -- Consumption_Signal/RConn1
  Generate_Consumption_Signal/RConn1 -- Order_OUT/RConn1
  sD1.9_Server/RConn1 -- Generate_Consumption_Signal/LConn1
  Order_IN/RConn1 -- sD1.9_Queue/LConn1
  sD1.9_Queue/RConn1 -- sD1.9_Server/LConn1

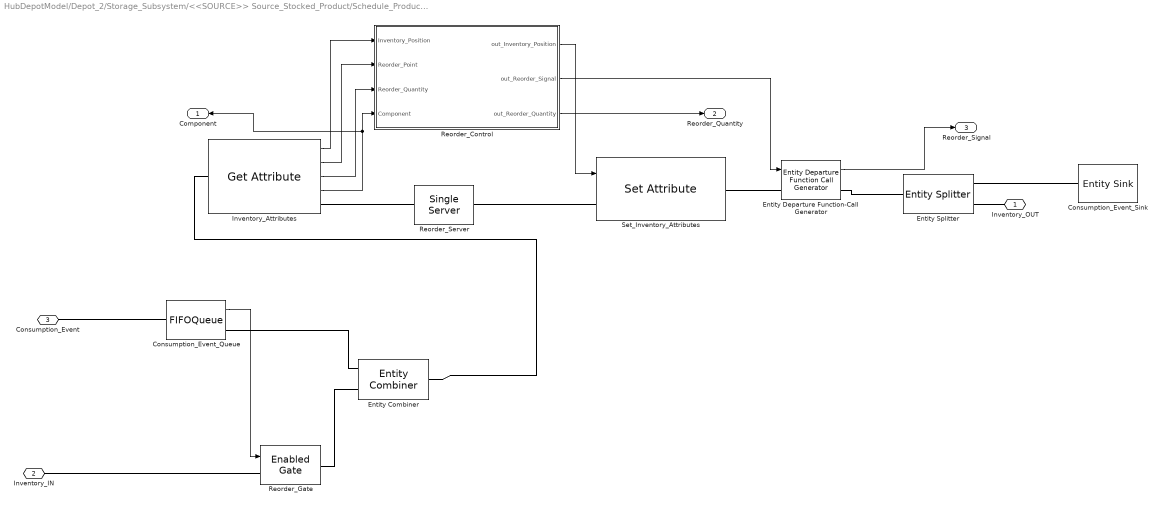
== system HubDepotModel/Depot_2/Storage_Subsystem/<<SOURCE>> Source_Stocked_Product/Schedule_Product_Deliveries_CONTROL ==
  Consumption_Event_Queue : FIFOQueue  StatNumberInBlock=on
      settings: OutputPortMap=o1
  Consumption_Event_Sink : EntitySink
  Entity Combiner : EntityCombiner  NumberInputPorts=2
  Entity Departure Function-Call Generator : EntityDepartureFunctionCallGenerator  EnableE1Port=on
  Entity Splitter : EntitySplitter  NumberOutputPorts=2
  Inventory_Attributes : GetAttribute  AttributeName=Inventory_Position|Reorder_Point|Reorder_Quantity|Component  AttributeMissing=Error|Error|Error|Error  AttributeDefaultValue=1|1|1|1  AttributeTreatAsVector=1|1|1|1  AttributeSendTiming=After entity departure|After entity departure|After entity departure|After entity departure  EvaluatedDefaultAttributeValue={[];[];[];[]}
      settings: OutputPortMap=o1,o2,o3,o4
  Reorder_Control : MATLAB Function  TreatAsAtomicUnit=on
  Reorder_Gate : EnabledGate
  Reorder_Server : SingleServer  ServiceTime=0
  Set_Inventory_Attributes : SetAttribute  AttributeName=Inventory_Position  AttributeFrom=Signal port  EvaluatedAttributeValue={[]}
  Inventory_OUT : PMIOPort  Port=1  Side=Right
  Inventory_IN : PMIOPort  Port=2  Side=Left
  Consumption_Event : PMIOPort  Port=3  Side=Left
  Component : Outport
  Reorder_Quantity : Outport  Port=2
  Reorder_Signal : Outport  Port=3
  wires:
  Entity Departure Function-Call Generator/1 -> Reorder_Signal/1
  Reorder_Control/3(out_Reorder_Quantity) -> Reorder_Quantity/1
  Consumption_Event_Queue/1 -> Reorder_Gate/1
  Reorder_Control/2(out_Reorder_Signal) -> Entity Departure Function-Call Generator/1
  Inventory_Attributes/4 -> Component/1, Reorder_Control/4(Component)
  Reorder_Control/1(out_Inventory_Position) -> Set_Inventory_Attributes/1
  Inventory_Attributes/3 -> Reorder_Control/3(Reorder_Quantity)
  Inventory_Attributes/2 -> Reorder_Control/2(Reorder_Point)
  Inventory_Attributes/1 -> Reorder_Control/1(Inventory_Position)
  connections:
  Entity Departure Function-Call Generator/RConn1 -- Entity Splitter/LConn1
  Set_Inventory_Attributes/RConn1 -- Entity Departure Function-Call Generator/LConn1
  Reorder_Server/RConn1 -- Set_Inventory_Attributes/LConn1
  Inventory_IN/RConn1 -- Reorder_Gate/LConn1
  Inventory_Attributes/RConn1 -- Reorder_Server/LConn1
  Inventory_OUT/RConn1 -- Entity Splitter/RConn2
  Entity Combiner/RConn1 -- Inventory_Attributes/LConn1
  Reorder_Gate/RConn1 -- Entity Combiner/LConn2
  Entity Splitter/RConn1 -- Consumption_Event_Sink/LConn1
  Consumption_Event_Queue/RConn1 -- Entity Combiner/LConn1
  Consumption_Event/RConn1 -- Consumption_Event_Queue/LConn1

== system HubDepotModel/Depot_2/Storage_Subsystem/<<SOURCE>> Source_Stocked_Product/Transfer_Product_CONTROL ==
  Calculate_Inventory : MATLAB Function  TreatAsAtomicUnit=on
  Combine_Inventory_and_Availability : EntityCombiner  NumberInputPorts=2
  FIFO Queue : FIFOQueue
  Inventory_Availability_Attributes : GetAttribute  AttributeName=Component|Shipment_Quantity|Net_Inventory  AttributeMissing=Error|Error|Error  AttributeDefaultValue=1|1|1  AttributeTreatAsVector=1|1|1  AttributeSendTiming=After entity departure|After entity departure|After entity departure  EvaluatedDefaultAttributeValue={[];[];[]}
      settings: OutputPortMap=o1,o2,o3
  Inventory_Availability_Sink : EntitySink
  Return_Inventory : EntitySplitter  NumberOutputPorts=2
  Server : SingleServer  ServiceTime=0
  Set_Inventory_Level : SetAttribute  AttributeName=Net_Inventory  AttributeFrom=Signal port  EvaluatedAttributeValue={[]}
  Inventory_OUT : PMIOPort  Port=1  Side=Right
  Inventory_IN : PMIOPort  Port=2  Side=Left
  Inventory_Availability_Signal : PMIOPort  Port=3  Side=Left
  wires:
  Inventory_Availability_Attributes/2 -> Calculate_Inventory/3(Shipment_Quantity)
  Inventory_Availability_Attributes/3 -> Calculate_Inventory/1(Net_Inventory)
  Calculate_Inventory/1(out_Inventory) -> Set_Inventory_Level/1
  Inventory_Availability_Attributes/1 -> Calculate_Inventory/2(Component)
  connections:
  Inventory_IN/RConn1 -- Combine_Inventory_and_Availability/LConn1
  FIFO Queue/RConn1 -- Combine_Inventory_and_Availability/LConn2
  Inventory_Availability_Signal/RConn1 -- FIFO Queue/LConn1
  Inventory_OUT/RConn1 -- Return_Inventory/RConn1
  Set_Inventory_Level/RConn1 -- Return_Inventory/LConn1
  Return_Inventory/RConn2 -- Inventory_Availability_Sink/LConn1
  Server/RConn1 -- Set_Inventory_Level/LConn1
  Inventory_Availability_Attributes/RConn1 -- Server/LConn1
  Combine_Inventory_and_Availability/RConn1 -- Inventory_Availability_Attributes/LConn1

== system HubDepotModel/Depot_2/Storage_Subsystem/<<SOURCE>> Source_Stocked_Product/sS1.1_Schedule_Product_Deliveries_PLANT ==
  Component : Inport
  Reorder_Quantity : Inport  Port=2
  Reorder_Signal : Inport  Port=3
  Generate_Procurement_Order : Subsystem
  Schedule_Product_Deliveries_Server : NServer  NumberOfServers=inf  ServiceTime=0
  Set_Procurement_Order : SetAttribute  AttributeName=Component|Order_Quantity|Supplier|Customer  AttributeFrom=Signal port|Signal port|Dialog|Dialog  AttributeValue=1|1|1|2  AttributeTreatAsVector=1|1|1|1  EvaluatedAttributeValue={[];[];1;2}
      settings: InputPortMap=u0,u1
  Procurement_Order : PMIOPort  Port=1  Side=Right
  wires:
  Reorder_Signal/1 -> Generate_Procurement_Order/1(Reorder_Signal)
  Reorder_Quantity/1 -> Set_Procurement_Order/2
  Component/1 -> Set_Procurement_Order/1
  connections:
  Procurement_Order/RConn1 -- Set_Procurement_Order/RConn1
  Schedule_Product_Deliveries_Server/RConn1 -- Set_Procurement_Order/LConn1
  Generate_Procurement_Order/RConn1 -- Schedule_Product_Deliveries_Server/LConn1

== system HubDepotModel/Depot_2/Storage_Subsystem/<<SOURCE>> Source_Stocked_Product/sS1.2_Receive_Product_PLANT ==
  sS1.2_Queue : FIFOQueue  Capacity=inf
  sS1.2_Server : NServer  NumberOfServers=inf  ServiceTime=0
  Shipment_IN : PMIOPort  Port=1  Side=Left
  Component_OUT : PMIOPort  Port=2  Side=Right
  connections:
  Component_OUT/RConn1 -- sS1.2_Server/RConn1
  Shipment_IN/RConn1 -- sS1.2_Queue/LConn1
  sS1.2_Queue/RConn1 -- sS1.2_Server/LConn1

== system HubDepotModel/Depot_2/Storage_Subsystem/<<SOURCE>> Source_Stocked_Product/sS1.3_Transfer_Product_PLANT ==
  sS1.4_Queue : FIFOQueue
  sS1.4_Server : NServer  NumberOfServers=inf  ServiceTime=0
  Component_IN : PMIOPort  Port=1  Side=Left
  Inventory_Availability_Signal : PMIOPort  Port=2  Side=Right
  connections:
  Inventory_Availability_Signal/RConn1 -- sS1.4_Server/RConn1
  Component_IN/RConn1 -- sS1.4_Queue/LConn1
  sS1.4_Queue/RConn1 -- sS1.4_Server/LConn1

== system HubDepotModel/Depot_2/Storage_Subsystem/<<SOURCE>> Source_Stocked_Product/sS1.3_Verify_Product_PLANT ==
  sS1.3_Queue : FIFOQueue  Capacity=inf
  sS1.3_Server : NServer  NumberOfServers=inf  ServiceTime=0
  Component_IN : PMIOPort  Port=1  Side=Left
  Component_OUT : PMIOPort  Port=2  Side=Right
  connections:
  Component_OUT/RConn1 -- sS1.3_Server/RConn1
  Component_IN/RConn1 -- sS1.3_Queue/LConn1
  sS1.3_Queue/RConn1 -- sS1.3_Server/LConn1

== system HubDepotModel/Depot_3/Storage_Subsystem/<<DELIVER>>Deliver_Stocked_Product/Deliver_Stocked_Product_CONTROL ==
  Calculate_Inventory_C : MATLAB Function  TreatAsAtomicUnit=on
  Combine_Consumption_Inventory : EntityCombiner  NumberInputPorts=2
  Consumption_Attributes : GetAttribute  AttributeName=Component|Consumption_Quantity|Net_Inventory|Inventory_Position  AttributeMissing=Error|Error|Error|Error  AttributeDefaultValue=1|1|1|1  AttributeTreatAsVector=1|1|1|1  AttributeSendTiming=After entity departure|After entity departure|After entity departure|After entity departure  EvaluatedDefaultAttributeValue={[];[];[];[]}
      settings: OutputPortMap=o1,o2,o3,o4
  Consumption_Server : SingleServer  ServiceTime=0
  Consumption_Sink : EntitySink
  FIFO Queue : FIFOQueue
  Replicate : Replicate  NumberOutputPorts=2
  Return_Inventory : EntitySplitter  NumberOutputPorts=2
  Set_Inventory_Level : SetAttribute  AttributeName=Net_Inventory|Inventory_Position  AttributeFrom=Signal port|Signal port  AttributeValue=1|1  AttributeTreatAsVector=1|1  EvaluatedAttributeValue={[];[]}
      settings: InputPortMap=u0,u1
  Inventory_IN : PMIOPort  Port=1  Side=Left
  Consumption_Signal_IN : PMIOPort  Port=2  Side=Left
  Consumption_Signal_OUT : PMIOPort  Port=3  Side=Right
  Inventory_OUT : PMIOPort  Port=4  Side=Right
  wires:
  Calculate_Inventory_C/2(out_Inventory_Position) -> Set_Inventory_Level/2
  Consumption_Attributes/4 -> Calculate_Inventory_C/2(Inventory_Position)
  Consumption_Attributes/2 -> Calculate_Inventory_C/4(Consumption_Quantity)
  Consumption_Attributes/3 -> Calculate_Inventory_C/1(Net_Inventory)
  Calculate_Inventory_C/1(out_Net_Inventory) -> Set_Inventory_Level/1
  Consumption_Attributes/1 -> Calculate_Inventory_C/3(Component)
  connections:
  Inventory_OUT/RConn1 -- Return_Inventory/RConn1
  Set_Inventory_Level/RConn1 -- Return_Inventory/LConn1
  Replicate/RConn2 -- Consumption_Signal_OUT/RConn1
  Return_Inventory/RConn2 -- Consumption_Sink/LConn1
  Consumption_Server/RConn1 -- Set_Inventory_Level/LConn1
  Consumption_Attributes/RConn1 -- Consumption_Server/LConn1
  Combine_Consumption_Inventory/RConn1 -- Consumption_Attributes/LConn1
  Replicate/RConn1 -- Combine_Consumption_Inventory/LConn2
  Inventory_IN/RConn1 -- Combine_Consumption_Inventory/LConn1
  Consumption_Signal_IN/RConn1 -- FIFO Queue/LConn1
  FIFO Queue/RConn1 -- Replicate/LConn1

== system HubDepotModel/Depot_3/Storage_Subsystem/<<DELIVER>>Deliver_Stocked_Product/sD1.10_Pack_Order_PLANT ==
  Entity Departure Function-Call Generator : EntityDepartureFunctionCallGenerator
  Event-Based Entity Generator : EventBasedEntityGenerator  GenerateEntitiesUpon=Function call from port fcn
  Get_Order_Attribute : GetAttribute  AttributeName=Component|Order_Quantity|Customer  AttributeMissing=Error|Error|Error  AttributeDefaultValue=1|1|1  AttributeTreatAsVector=1|1|1  AttributeSendTiming=After entity departure|After entity departure|After entity departure  EvaluatedDefaultAttributeValue={[];[];[]}
      settings: OutputPortMap=o1,o2,o3
  Order_Sink : EntitySink
  Set_Shipment_Attributes : SetAttribute  AttributeName=Component|Shipment_Quantity|Customer  AttributeFrom=Signal port|Signal port|Signal port  AttributeValue=1|1|1  AttributeTreatAsVector=1|1|1  EvaluatedAttributeValue={[];[];[]}
      settings: InputPortMap=u0,u1,u2
  sD1.10_Queue : FIFOQueue
  sD1.10_Server : NServer  NumberOfServers=inf  ServiceTime=0
  Order_IN : PMIOPort  Port=1  Side=Left
  Shipment_OUT : PMIOPort  Port=2  Side=Right
  wires:
  Get_Order_Attribute/3 -> Set_Shipment_Attributes/3
  Get_Order_Attribute/1 -> Set_Shipment_Attributes/1
  Get_Order_Attribute/2 -> Set_Shipment_Attributes/2
  Entity Departure Function-Call Generator/1 -> Event-Based Entity Generator/1
  connections:
  Get_Order_Attribute/RConn1 -- Entity Departure Function-Call Generator/LConn1
  sD1.10_Server/RConn1 -- Get_Order_Attribute/LConn1
  Order_Sink/LConn1 -- Entity Departure Function-Call Generator/RConn1
  Set_Shipment_Attributes/RConn1 -- Shipment_OUT/RConn1
  Event-Based Entity Generator/RConn1 -- Set_Shipment_Attributes/LConn1
  Order_IN/RConn1 -- sD1.10_Queue/LConn1
  sD1.10_Queue/RConn1 -- sD1.10_Server/LConn1

== system HubDepotModel/Depot_3/Storage_Subsystem/<<DELIVER>>Deliver_Stocked_Product/sD1.11_Load_Order_PLANT ==
  sD1.11_Queue : FIFOQueue
  sD1.11_Server : NServer  NumberOfServers=inf  ServiceTime=0
  Shipment_IN : PMIOPort  Port=1  Side=Left
  Shipment_OUT : PMIOPort  Port=2  Side=Right
  connections:
  Shipment_OUT/RConn1 -- sD1.11_Server/RConn1
  Shipment_IN/RConn1 -- sD1.11_Queue/LConn1
  sD1.11_Queue/RConn1 -- sD1.11_Server/LConn1

== system HubDepotModel/Depot_3/Storage_Subsystem/<<DELIVER>>Deliver_Stocked_Product/sD1.2_Receive_Order_PLANT ==
  sD1.2_Queue : FIFOQueue
  sD1.2_Server : NServer  NumberOfServers=inf  ServiceTime=0
  Order_IN : PMIOPort  Port=1  Side=Left
  Order_OUT : PMIOPort  Port=2  Side=Right
  connections:
  Order_OUT/RConn1 -- sD1.2_Server/RConn1
  Order_IN/RConn1 -- sD1.2_Queue/LConn1
  sD1.2_Queue/RConn1 -- sD1.2_Server/LConn1

== system HubDepotModel/Depot_3/Storage_Subsystem/<<DELIVER>>Deliver_Stocked_Product/sD1.4_Consolidate_Orders_PLANT ==
  sD1.4_Queue : FIFOQueue
  sD1.4_Server : NServer  NumberOfServers=inf  ServiceTime=0
  Order_IN : PMIOPort  Port=1  Side=Left
  Order_OUT : PMIOPort  Port=2  Side=Right
  connections:
  Order_OUT/RConn1 -- sD1.4_Server/RConn1
  Order_IN/RConn1 -- sD1.4_Queue/LConn1
  sD1.4_Queue/RConn1 -- sD1.4_Server/LConn1

== system HubDepotModel/Depot_3/Storage_Subsystem/<<DELIVER>>Deliver_Stocked_Product/sD1.9_Pick_Order_PLANT ==
  Generate_Consumption_Signal : Subsystem
  sD1.9_Queue : FIFOQueue
  sD1.9_Server : NServer  NumberOfServers=inf  ServiceTime=0
  Order_IN : PMIOPort  Port=1  Side=Left
  Consumption_Signal : PMIOPort  Port=2  Side=Right
  Order_OUT : PMIOPort  Port=3  Side=Right
  connections:
  Generate_Consumption_Signal/RConn2 -- Consumption_Signal/RConn1
  Generate_Consumption_Signal/RConn1 -- Order_OUT/RConn1
  sD1.9_Server/RConn1 -- Generate_Consumption_Signal/LConn1
  Order_IN/RConn1 -- sD1.9_Queue/LConn1
  sD1.9_Queue/RConn1 -- sD1.9_Server/LConn1

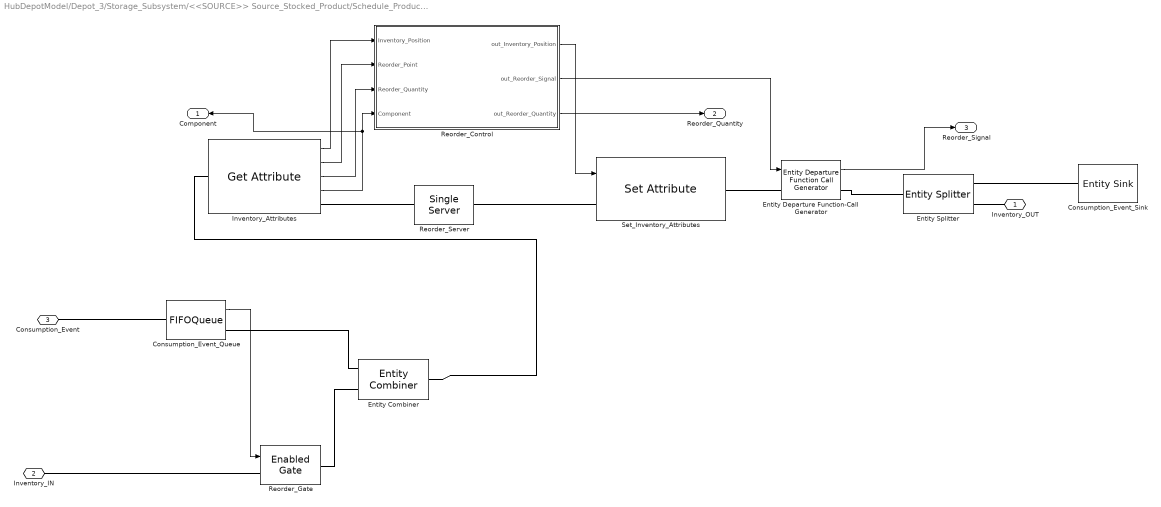
== system HubDepotModel/Depot_3/Storage_Subsystem/<<SOURCE>> Source_Stocked_Product/Schedule_Product_Deliveries_CONTROL ==
  Consumption_Event_Queue : FIFOQueue  StatNumberInBlock=on
      settings: OutputPortMap=o1
  Consumption_Event_Sink : EntitySink
  Entity Combiner : EntityCombiner  NumberInputPorts=2
  Entity Departure Function-Call Generator : EntityDepartureFunctionCallGenerator  EnableE1Port=on
  Entity Splitter : EntitySplitter  NumberOutputPorts=2
  Inventory_Attributes : GetAttribute  AttributeName=Inventory_Position|Reorder_Point|Reorder_Quantity|Component  AttributeMissing=Error|Error|Error|Error  AttributeDefaultValue=1|1|1|1  AttributeTreatAsVector=1|1|1|1  AttributeSendTiming=After entity departure|After entity departure|After entity departure|After entity departure  EvaluatedDefaultAttributeValue={[];[];[];[]}
      settings: OutputPortMap=o1,o2,o3,o4
  Reorder_Control : MATLAB Function  TreatAsAtomicUnit=on
  Reorder_Gate : EnabledGate
  Reorder_Server : SingleServer  ServiceTime=0
  Set_Inventory_Attributes : SetAttribute  AttributeName=Inventory_Position  AttributeFrom=Signal port  EvaluatedAttributeValue={[]}
  Inventory_OUT : PMIOPort  Port=1  Side=Right
  Inventory_IN : PMIOPort  Port=2  Side=Left
  Consumption_Event : PMIOPort  Port=3  Side=Left
  Component : Outport
  Reorder_Quantity : Outport  Port=2
  Reorder_Signal : Outport  Port=3
  wires:
  Entity Departure Function-Call Generator/1 -> Reorder_Signal/1
  Reorder_Control/3(out_Reorder_Quantity) -> Reorder_Quantity/1
  Consumption_Event_Queue/1 -> Reorder_Gate/1
  Reorder_Control/2(out_Reorder_Signal) -> Entity Departure Function-Call Generator/1
  Inventory_Attributes/4 -> Component/1, Reorder_Control/4(Component)
  Reorder_Control/1(out_Inventory_Position) -> Set_Inventory_Attributes/1
  Inventory_Attributes/3 -> Reorder_Control/3(Reorder_Quantity)
  Inventory_Attributes/2 -> Reorder_Control/2(Reorder_Point)
  Inventory_Attributes/1 -> Reorder_Control/1(Inventory_Position)
  connections:
  Entity Departure Function-Call Generator/RConn1 -- Entity Splitter/LConn1
  Set_Inventory_Attributes/RConn1 -- Entity Departure Function-Call Generator/LConn1
  Reorder_Server/RConn1 -- Set_Inventory_Attributes/LConn1
  Inventory_IN/RConn1 -- Reorder_Gate/LConn1
  Inventory_Attributes/RConn1 -- Reorder_Server/LConn1
  Inventory_OUT/RConn1 -- Entity Splitter/RConn2
  Entity Combiner/RConn1 -- Inventory_Attributes/LConn1
  Reorder_Gate/RConn1 -- Entity Combiner/LConn2
  Entity Splitter/RConn1 -- Consumption_Event_Sink/LConn1
  Consumption_Event_Queue/RConn1 -- Entity Combiner/LConn1
  Consumption_Event/RConn1 -- Consumption_Event_Queue/LConn1
